simulink library "ThetaOverFlowFilter"  (R2016b)
settings: Solver=VariableStepAuto  StartTime=0.0  StopTime=10.0  RelTol=1e-3
settings Model: Creator=oelkawok  LastModifiedBy=oelkawok

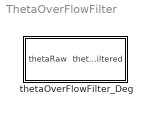
== system ThetaOverFlowFilter ==
  thetaOverFlowFilter_Deg : Subsystem

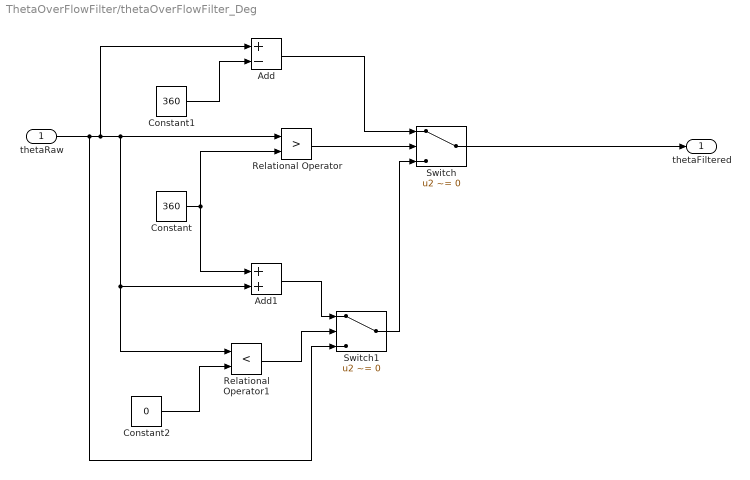
== system ThetaOverFlowFilter/thetaOverFlowFilter_Deg ==
  thetaRaw : Inport
  Add : Sum  Inputs=+-
  Add1 : Sum
  Constant : Constant  Value=360
  Constant1 : Constant  Value=360
  Constant2 : Constant  Value=0
  Relational Operator : RelationalOperator  Operator=>  OutDataTypeStr=boolean  RndMeth=Nearest
  Relational Operator1 : RelationalOperator  Operator=<  OutDataTypeStr=boolean  RndMeth=Nearest
  Switch : Switch  Criteria=u2 ~= 0
  Switch1 : Switch  Criteria=u2 ~= 0
  thetaFiltered : Outport
  wires:
  thetaRaw/1 -> Switch1/3, Add/1, Add1/2, Relational Operator1/1, Relational Operator/1
  Constant/1 -> Add1/1, Relational Operator/2
  Relational Operator/1 -> Switch/2
  Constant1/1 -> Add/2
  Add/1 -> Switch/1
  Constant2/1 -> Relational Operator1/2
  Relational Operator1/1 -> Switch1/2
  Add1/1 -> Switch1/1
  Switch1/1 -> Switch/3
  Switch/1 -> thetaFiltered/1
